simulink library "lib_polar_to_cart_coor_transformer"  (R2023a)
settings: Solver=VariableStepAuto  StartTime=0.0  StopTime=10.0  RelTol=1e-3
libraries: lib_conversion x4, vhit_control_library x2
settings Model: Creator=cav2ofo  LastModifiedBy=lenovo
settings OptimizationCC: ReuseModelBlockBuffer=off

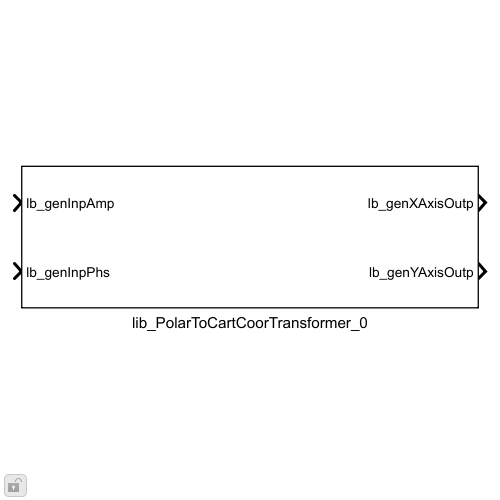
[thumbnail: Simulink's stored preview of the top-level diagram]
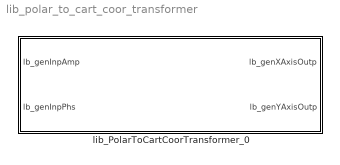
== system lib_polar_to_cart_coor_transformer ==
  lib_PolarToCartCoorTransformer_0 : Subsystem  mask{lb_parLktSize=1024, lb_parOutpDataType=Inherit: Inherit via back propagation}
      mask prompts: lb_parLktSize "Lookup table size:"; lb_parOutpDataType "Outputs data type:"
      mask init:
      | lb_parLktSizeNum = str2double(lb_parLktSize);
      mask TypeOptions lb_parLktSize: 128 | 256 | 512 | 1024 | 2048
      mask DialogControl DescGroupVar Prompt: VHIT control library
      mask DialogControl DescTextVar Prompt: Polar to cartesian coordinates transformer
      mask DialogControl Container3 Prompt: Data type

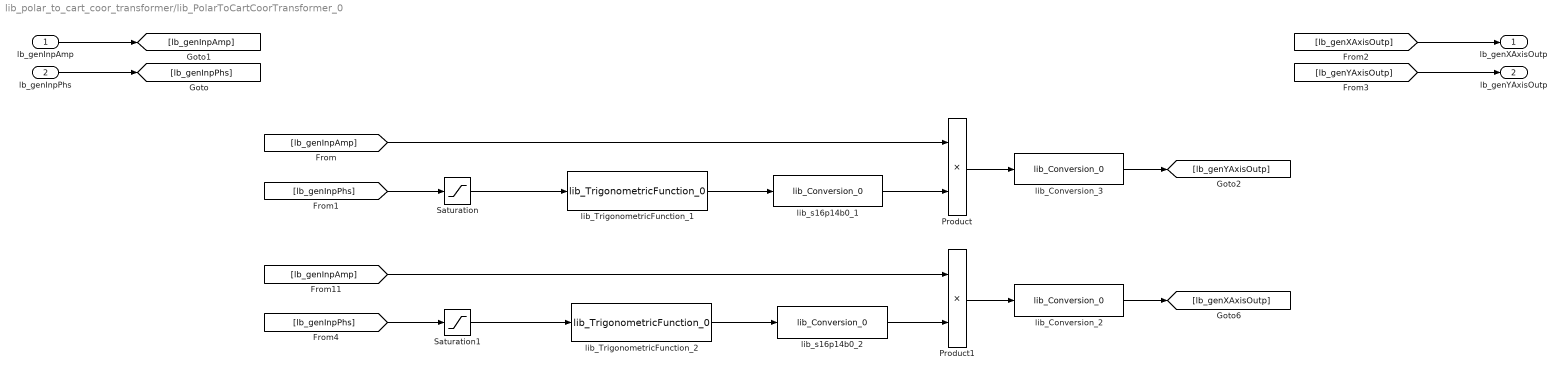
== system lib_polar_to_cart_coor_transformer/lib_PolarToCartCoorTransformer_0 ==
  lb_genInpAmp : Inport
  lb_genInpPhs : Inport  Port=2
  Product : Product  OutDataTypeStr=Inherit: Inherit via back propagation
  Product1 : Product  OutDataTypeStr=Inherit: Inherit via back propagation
  Saturation : Saturate  UpperLimit=2*pi  LowerLimit=0
  Saturation1 : Saturate  UpperLimit=2*pi  LowerLimit=0
  lib_Conversion_2 : lib_conversion/lib_Conversion_0  lb_parDataType=lb_parOutpDataType  lb_parOutpMaxVal=[]  lb_parOutpMinVal=[]  lb_parSatFlag=off
  lib_Conversion_3 : lib_conversion/lib_Conversion_0  lb_parDataType=lb_parOutpDataType  lb_parOutpMaxVal=[]  lb_parOutpMinVal=[]  lb_parSatFlag=off
  lib_TrigonometricFunction_1 : vhit_control_library/lib_TrigonometricFunction_0  lb_parSelSigType=Sine  lb_parLktSizeStr=1024  lb_parOutpDataType=Inherit: Inherit via back propagation
  lib_TrigonometricFunction_2 : vhit_control_library/lib_TrigonometricFunction_0  lb_parSelSigType=Cosine  lb_parLktSizeStr=1024  lb_parOutpDataType=Inherit: Inherit via back propagation
  lib_s16p14b0_1 : lib_conversion/lib_Conversion_0  lb_parDataType=fixdt(1,16,2^-14,0)  lb_parOutpMaxVal=[]  lb_parOutpMinVal=[]  lb_parSatFlag=off
  lib_s16p14b0_2 : lib_conversion/lib_Conversion_0  lb_parDataType=fixdt(1,16,2^-14,0)  lb_parOutpMaxVal=[]  lb_parOutpMinVal=[]  lb_parSatFlag=off
  lb_genXAxisOutp : Outport
  lb_genYAxisOutp : Outport  Port=2
  wires:
  Saturation1/1 -> lib_TrigonometricFunction_2/1
  [lb_genInpPhs] -> Saturation1/1
  lib_Conversion_2/1 -> [lb_genXAxisOutp]
  Product1/1 -> lib_Conversion_2/1
  [lb_genInpAmp] -> Product1/1
  lib_s16p14b0_2/1 -> Product1/2
  lib_TrigonometricFunction_2/1 -> lib_s16p14b0_2/1
  lib_s16p14b0_1/1 -> Product/2
  lib_Conversion_3/1 -> [lb_genYAxisOutp]
  Product/1 -> lib_Conversion_3/1
  [lb_genInpAmp] -> Product/1
  lib_TrigonometricFunction_1/1 -> lib_s16p14b0_1/1
  Saturation/1 -> lib_TrigonometricFunction_1/1
  [lb_genInpPhs] -> Saturation/1
  [lb_genYAxisOutp] -> lb_genYAxisOutp/1
  [lb_genXAxisOutp] -> lb_genXAxisOutp/1
  lb_genInpAmp/1 -> [lb_genInpAmp]
  lb_genInpPhs/1 -> [lb_genInpPhs]
